simulink model "Snapbot_6leg"  (R2020a)
settings: Solver=FixedStepAuto  StartTime=0.0  StopTime=20  FixedStep=0.001  RelTol=1e-3
PreLoadFcn:
  | startup_Contact_Forces;
InitFcn:
  | SnapbotParameters_6leg;
StopFcn:
  | snapbot_plot;
model workspace (MATLAB code in the model file):
  | % Simscape(TM) Multibody(TM) version: 7.0
  | 
  | % This is a model data file derived from a Simscape Multibody Import XML file using the smimport function.
  | % The data in this file sets the block parameter values in an imported Simscape Multibody model.
  | % For more information on this file, see the smimport function help page in the Simscape Multibody documentation.
  | % You can modify numerical values, but avoid any other changes to this file.
  | % Do not add code to this file. Do not edit the physical units shown in comments.
  | 
  | %%%VariableName:smiData
  | 
  | 
  | %============= RigidTransform =============%
  | 
  | %Initialize the RigidTransform structure array by filling in null values.
  | smiData.RigidTransform(41).translation = [0.0 0.0 0.0];
  | smiData.RigidTransform(41).angle = 0.0;
  | smiData.RigidTransform(41).axis = [0.0 0.0 0.0];
  | smiData.RigidTransform(41).ID = '';
  | 
  | %Translation Method - Cartesian
  | %Rotation Method - Arbitrary Axis
  | smiData.RigidTransform(1).translation = [0 0 3.5000000000000031];  % mm
  | smiData.RigidTransform(1).angle = 0;  % rad
  | smiData.RigidTransform(1).axis = [0 0 0];
  | smiData.RigidTransform(1).ID = 'B[Leg_Assembly_Y-P:Leg_part_01_yaw-1:-:Leg_Assembly_Y-P:v4_Hyb_X-430_IDLE_uncut-1]';
  | 
  | %Translation Method - Cartesian
  | %Rotation Method - Arbitrary Axis
  | smiData.RigidTransform(2).translation = [1.7377765892945298e-13 -35.249999999999865 -4.1211478674085811e-13];  % mm
  | smiData.RigidTransform(2).angle = 3.1415926535897931;  % rad
  | smiData.RigidTransform(2).axis = [3.9252311467098009e-17 -0.70710678118654757 -0.70710678118654746];
  | smiData.RigidTransform(2).ID = 'F[Leg_Assembly_Y-P:Leg_part_01_yaw-1:-:Leg_Assembly_Y-P:v4_Hyb_X-430_IDLE_uncut-1]';
  | 
  | %Translation Method - Cartesian
  | %Rotation Method - Arbitrary Axis
  | smiData.RigidTransform(3).translation = [18.999999999999996 0 -21.500000000000004];  % mm
  | smiData.RigidTransform(3).angle = 2.0943951023931957;  % rad
  | smiData.RigidTransform(3).axis = [0.57735026918962562 0.57735026918962584 0.57735026918962584];
  | smiData.RigidTransform(3).ID = 'B[Leg_Assembly_Y-P:Leg_part_02_Yaw-1:-:Leg_Assembly_Y-P:v4_Hyb_X-430_IDLE_uncut-1]';
  | 
  | %Translation Method - Cartesian
  | %Rotation Method - Arbitrary Axis
  | smiData.RigidTransform(4).translation = [-2.7613467068476893e-12 6.9988459472369868e-13 19];  % mm
  | smiData.RigidTransform(4).angle = 4.7102773760513248e-16;  % rad
  | smiData.RigidTransform(4).axis = [-0.94280904158206347 0.3333333333333332 -7.4014868308343741e-17];
  | smiData.RigidTransform(4).ID = 'F[Leg_Assembly_Y-P:Leg_part_02_Yaw-1:-:Leg_Assembly_Y-P:v4_Hyb_X-430_IDLE_uncut-1]';
  | 
  | %Translation Method - Cartesian
  | %Rotation Method - Arbitrary Axis
  | smiData.RigidTransform(5).translation = [8.3000000000000025 6.0000000000000009 -1.5000000000000013];  % mm
  | smiData.RigidTransform(5).angle = 3.1415926535897931;  % rad
  | smiData.RigidTransform(5).axis = [1 0 0];
  | smiData.RigidTransform(5).ID = 'B[Leg_Assembly_Y-P:Leg_part_02_Yaw-1:-:Leg_Assembly_Y-P:v4_Hyb_X-430_IDLE_uncut-2]';
  | 
  | %Translation Method - Cartesian
  | %Rotation Method - Arbitrary Axis
  | smiData.RigidTransform(6).translation = [-8.0000000000000853 -36.749999999999993 6.0000000000000142];  % mm
  | smiData.RigidTransform(6).angle = 3.1415926535897931;  % rad
  | smiData.RigidTransform(6).axis = [5.5511151231257827e-17 0.70710678118654757 -0.70710678118654746];
  | smiData.RigidTransform(6).ID = 'F[Leg_Assembly_Y-P:Leg_part_02_Yaw-1:-:Leg_Assembly_Y-P:v4_Hyb_X-430_IDLE_uncut-2]';
  | 
  | %Translation Method - Cartesian
  | %Rotation Method - Arbitrary Axis
  | smiData.RigidTransform(7).translation = [-5.7500000000000053 17.749999999999996 20.999999999999993];  % mm
  | smiData.RigidTransform(7).angle = 2.0943951023931953;  % rad
  | smiData.RigidTransform(7).axis = [0.57735026918962584 -0.57735026918962584 0.57735026918962584];
  | smiData.RigidTransform(7).ID = 'B[Leg_Assembly_Y-P:Leg_part_03-1:-:Leg_Assembly_Y-P:v4_Hyb_X-430_IDLE_uncut-2]';
  | 
  | %Translation Method - Cartesian
  | %Rotation Method - Arbitrary Axis
  | smiData.RigidTransform(8).translation = [-17.75000000000005 -4.0000000000015383 6.000000000000135];  % mm
  | smiData.RigidTransform(8).angle = 2.0943951023931953;  % rad
  | smiData.RigidTransform(8).axis = [0.57735026918962562 0.57735026918962584 0.57735026918962595];
  | smiData.RigidTransform(8).ID = 'F[Leg_Assembly_Y-P:Leg_part_03-1:-:Leg_Assembly_Y-P:v4_Hyb_X-430_IDLE_uncut-2]';
  | 
  | %Translation Method - Cartesian
  | %Rotation Method - Arbitrary Axis
  | smiData.RigidTransform(9).translation = [47.999999999999986 0 0];  % mm
  | smiData.RigidTransform(9).angle = 2.0943951023931953;  % rad
  | smiData.RigidTransform(9).axis = [-0.57735026918962584 -0.57735026918962584 0.57735026918962584];
  | smiData.RigidTransform(9).ID = 'B[Leg_Assembly_Y-P:Leg_part_04-1:-:Leg_Assembly_Y-P:v4_Hyb_X-430_IDLE_uncut-2]';
  | 
  | %Translation Method - Cartesian
  | %Rotation Method - Arbitrary Axis
  | smiData.RigidTransform(10).translation = [-1.2789769243681803e-12 1.5383250229206169e-12 24.000000000000025];  % mm
  | smiData.RigidTransform(10).angle = 3.1415926535897931;  % rad
  | smiData.RigidTransform(10).axis = [1 2.1382117680737565e-50 2.7755575615628914e-17];
  | smiData.RigidTransform(10).ID = 'F[Leg_Assembly_Y-P:Leg_part_04-1:-:Leg_Assembly_Y-P:v4_Hyb_X-430_IDLE_uncut-2]';
  | 
  | %Translation Method - Cartesian
  | %Rotation Method - Arbitrary Axis
  | smiData.RigidTransform(11).translation = [21.999999999999993 6.0000000000000053 -15.000000000000004];  % mm
  | smiData.RigidTransform(11).angle = 0;  % rad
  | smiData.RigidTransform(11).axis = [0 0 0];
  | smiData.RigidTransform(11).ID = 'B[Leg_Assembly_Y-P:Leg_part_03-1:-:Leg_Assembly_Y-P:Leg_part_06-1]';
  | 
  | %Translation Method - Cartesian
  | %Rotation Method - Arbitrary Axis
  | smiData.RigidTransform(12).translation = [-25.499999999999993 -6.4730443227745127e-12 -47.429999999998479];  % mm
  | smiData.RigidTransform(12).angle = 2.0943951023931953;  % rad
  | smiData.RigidTransform(12).axis = [0.57735026918962584 0.57735026918962584 0.57735026918962584];
  | smiData.RigidTransform(12).ID = 'F[Leg_Assembly_Y-P:Leg_part_03-1:-:Leg_Assembly_Y-P:Leg_part_06-1]';
  | 
  | %Translation Method - Cartesian
  | %Rotation Method - Arbitrary Axis
  | smiData.RigidTransform(13).translation = [18.500000000000004 0 0];  % mm
  | smiData.RigidTransform(13).angle = 2.0943951023931957;  % rad
  | smiData.RigidTransform(13).axis = [-0.57735026918962584 -0.57735026918962573 0.57735026918962573];
  | smiData.RigidTransform(13).ID = 'B[Leg_Assembly_Y-P:Leg_part_05-1:-:Leg_Assembly_Y-P:Leg_part_04-1]';
  | 
  | %Translation Method - Cartesian
  | %Rotation Method - Arbitrary Axis
  | smiData.RigidTransform(14).translation = [5.4999999999999645 -6.1227943166086393e-12 -59.999999999989711];  % mm
  | smiData.RigidTransform(14).angle = 2.0943951023931953;  % rad
  | smiData.RigidTransform(14).axis = [0.57735026918962584 0.57735026918962584 0.57735026918962584];
  | smiData.RigidTransform(14).ID = 'F[Leg_Assembly_Y-P:Leg_part_05-1:-:Leg_Assembly_Y-P:Leg_part_04-1]';
  | 
  | %Translation Method - Cartesian
  | %Rotation Method - Arbitrary Axis
  | smiData.RigidTransform(15).translation = [-4.5000000000000009 25 0];  % mm
  | smiData.RigidTransform(15).angle = 2.0943951023931953;  % rad
  | smiData.RigidTransform(15).axis = [-0.57735026918962584 -0.57735026918962584 0.57735026918962584];
  | smiData.RigidTransform(15).ID = 'B[Leg_Assembly_Y-P:Leg_part_05-1:-:Leg_Assembly_Y-P:Leg_part_06-1]';
  | 
  | %Translation Method - Cartesian
  | %Rotation Method - Arbitrary Axis
  | smiData.RigidTransform(16).translation = [8.9999999999998792 1.925328508647566e-12 -7.783518711315191e-13];  % mm
  | smiData.RigidTransform(16).angle = 2.0943951023931957;  % rad
  | smiData.RigidTransform(16).axis = [0.57735026918962584 0.57735026918962584 0.57735026918962562];
  | smiData.RigidTransform(16).ID = 'F[Leg_Assembly_Y-P:Leg_part_05-1:-:Leg_Assembly_Y-P:Leg_part_06-1]';
  | 
  | %Translation Method - Cartesian
  | %Rotation Method - Arbitrary Axis
  | smiData.RigidTransform(17).translation = [-29.14813879243771 31.324765133364547 -50.486057334570816];  % mm
  | smiData.RigidTransform(17).angle = 0.85969556486762932;  % rad
  | smiData.RigidTransform(17).axis = [-0.88342402684813537 0.43430848851138709 -0.17589236934665334];
  | smiData.RigidTransform(17).ID = 'B[Body_Frame-2:-:cover_IMU-1]';
  | 
  | %Translation Method - Cartesian
  | %Rotation Method - Arbitrary Axis
  | smiData.RigidTransform(18).translation = [-29.148138792437663 -3.675234866635499 -50.486057334570852];  % mm
  | smiData.RigidTransform(18).angle = 0.85969556486762932;  % rad
  | smiData.RigidTransform(18).axis = [-0.88342402684813526 0.43430848851138698 -0.17589236934665331];
  | smiData.RigidTransform(18).ID = 'F[Body_Frame-2:-:cover_IMU-1]';
  | 
  | %Translation Method - Cartesian
  | %Rotation Method - Arbitrary Axis
  | smiData.RigidTransform(19).translation = [-60.000000000000043 24.02083948120934 0];  % mm
  | smiData.RigidTransform(19).angle = 2.5346467848844187;  % rad
  | smiData.RigidTransform(19).axis = [-0.31314561301497384 -0.67154293423781708 0.67154293423781863];
  | smiData.RigidTransform(19).ID = 'B[Body_Frame-2:-:Leg_Assembly_Y-P-5:Leg_part_01_yaw-1]';
  | 
  | %Translation Method - Cartesian
  | %Rotation Method - Arbitrary Axis
  | smiData.RigidTransform(20).translation = [3.7154631030277672e-13 16.020839481209393 -21.000000000000213];  % mm
  | smiData.RigidTransform(20).angle = 1.6880425449503949;  % rad
  | smiData.RigidTransform(20).axis = [0.32361557711818967 -0.32361557711818179 0.88912649071598759];
  | smiData.RigidTransform(20).ID = 'F[Body_Frame-2:-:Leg_Assembly_Y-P-5:Leg_part_01_yaw-1]';
  | 
  | %Translation Method - Cartesian
  | %Rotation Method - Arbitrary Axis
  | smiData.RigidTransform(21).translation = [-17.984370389093243 16.010419740604632 -58.898751217406307];  % mm
  | smiData.RigidTransform(21).angle = 2.5668813081404753;  % rad
  | smiData.RigidTransform(21).axis = [-0.54469904781872214 -0.67552162020226258 0.49696427230203144];
  | smiData.RigidTransform(21).ID = 'B[Body_Frame-2:-:Leg_Assembly_Y-P-4:Leg_part_01_yaw-1]';
  | 
  | %Translation Method - Cartesian
  | %Rotation Method - Arbitrary Axis
  | smiData.RigidTransform(22).translation = [-13.874453980679904 8.0104197406047888 -21.000000000000171];  % mm
  | smiData.RigidTransform(22).angle = 1.5933089052267559;  % rad
  | smiData.RigidTransform(22).axis = [0.45474157432660411 0.14837486987203785 0.87817708838788178];
  | smiData.RigidTransform(22).ID = 'F[Body_Frame-2:-:Leg_Assembly_Y-P-4:Leg_part_01_yaw-1]';
  | 
  | %Translation Method - Cartesian
  | %Rotation Method - Arbitrary Axis
  | smiData.RigidTransform(23).translation = [0 50 0];  % mm
  | smiData.RigidTransform(23).angle = 2.0943951023931953;  % rad
  | smiData.RigidTransform(23).axis = [-0.57735026918962584 -0.57735026918962584 -0.57735026918962584];
  | smiData.RigidTransform(23).ID = 'B[floor-1:-:]';
  | 
  | %Translation Method - Cartesian
  | %Rotation Method - Arbitrary Axis
  | smiData.RigidTransform(24).translation = [0 -7.1054273576010019e-15 0];  % mm
  | smiData.RigidTransform(24).angle = 3.1415926535897931;  % rad
  | smiData.RigidTransform(24).axis = [0.70710678118654757 0.70710678118654757 -5.5511151231257839e-17];
  | smiData.RigidTransform(24).ID = 'F[floor-1:-:]';
  | 
  | %Translation Method - Cartesian
  | %Rotation Method - Arbitrary Axis
  | smiData.RigidTransform(25).translation = [29.999999999999982 24.02083948120934 -51.961524227066384];  % mm
  | smiData.RigidTransform(25).angle = 2.3875525638501713;  % rad
  | smiData.RigidTransform(25).axis = [0.97769691900991618 0.078837114487629617 0.19466238449629064];
  | smiData.RigidTransform(25).ID = 'B[Body_Frame-2:-:Leg_Assembly_Y-P-3:Leg_part_01_yaw-1]';
  | 
  | %Translation Method - Cartesian
  | %Rotation Method - Arbitrary Axis
  | smiData.RigidTransform(26).translation = [-4.3698378249246161e-13 16.020839481209286 -20.999999999999972];  % mm
  | smiData.RigidTransform(26).angle = 2.8078721686781996;  % rad
  | smiData.RigidTransform(26).axis = [0.061302152168850967 -0.34137689046920633 0.93792529808777547];
  | smiData.RigidTransform(26).ID = 'F[Body_Frame-2:-:Leg_Assembly_Y-P-3:Leg_part_01_yaw-1]';
  | 
  | %Translation Method - Cartesian
  | %Rotation Method - Arbitrary Axis
  | smiData.RigidTransform(27).translation = [30.000000000000536 24.02083948120934 51.961524227066057];  % mm
  | smiData.RigidTransform(27).angle = 0.85969556486763532;  % rad
  | smiData.RigidTransform(27).axis = [0.88342402684813182 0.43430848851139292 0.17589236934665639];
  | smiData.RigidTransform(27).ID = 'B[Body_Frame-2:-:Leg_Assembly_Y-P-2:Leg_part_01_yaw-1]';
  | 
  | %Translation Method - Cartesian
  | %Rotation Method - Arbitrary Axis
  | smiData.RigidTransform(28).translation = [5.6843418860808015e-14 16.020839481209322 -21.000000000000114];  % mm
  | smiData.RigidTransform(28).angle = 0.7800553012765955;  % rad
  | smiData.RigidTransform(28).axis = [0.88538441591605921 -0.15899134272919926 0.43682512403723389];
  | smiData.RigidTransform(28).ID = 'F[Body_Frame-2:-:Leg_Assembly_Y-P-2:Leg_part_01_yaw-1]';
  | 
  | %Translation Method - Cartesian
  | %Rotation Method - Arbitrary Axis
  | smiData.RigidTransform(29).translation = [0 16.020839481209414 -20.999999999999996];  % mm
  | smiData.RigidTransform(29).angle = 2.4434609527920594;  % rad
  | smiData.RigidTransform(29).axis = [-1 -2.3686015843339707e-16 6.5076793686420059e-16];
  | smiData.RigidTransform(29).ID = 'B[Leg_Assembly_Y-P-1:Leg_part_01_yaw-1:-:Body_Frame-2]';
  | 
  | %Translation Method - Cartesian
  | %Rotation Method - Arbitrary Axis
  | smiData.RigidTransform(30).translation = [-29.999999999999154 24.020839481209457 51.961524227066796];  % mm
  | smiData.RigidTransform(30).angle = 2.4682098215588208;  % rad
  | smiData.RigidTransform(30).axis = [-0.96166828182989805 -0.093787209197188054 -0.25767823950294];
  | smiData.RigidTransform(30).ID = 'F[Leg_Assembly_Y-P-1:Leg_part_01_yaw-1:-:Body_Frame-2]';
  | 
  | %Translation Method - Cartesian
  | %Rotation Method - Arbitrary Axis
  | smiData.RigidTransform(31).translation = [58.296277584874844 -3.6752348666354435 0];  % mm
  | smiData.RigidTransform(31).angle = 1.750366012803156;  % rad
  | smiData.RigidTransform(31).axis = [0.83481712947898612 0.38928162063502714 0.38928162063502642];
  | smiData.RigidTransform(31).ID = 'B[cover-2:-:Body_Frame-2]';
  | 
  | %Translation Method - Cartesian
  | %Rotation Method - Arbitrary Axis
  | smiData.RigidTransform(32).translation = [-58.296277584874161 -15.324765133364131 2.3909763058327371e-12];  % mm
  | smiData.RigidTransform(32).angle = 2.534646784884413;  % rad
  | smiData.RigidTransform(32).axis = [0.31314561301496746 -0.67154293423781519 -0.67154293423782341];
  | smiData.RigidTransform(32).ID = 'F[cover-2:-:Body_Frame-2]';
  | 
  | %Translation Method - Cartesian
  | %Rotation Method - Arbitrary Axis
  | smiData.RigidTransform(33).translation = [60.000000000000043 24.02083948120934 0];  % mm
  | smiData.RigidTransform(33).angle = 1.7503660128031577;  % rad
  | smiData.RigidTransform(33).axis = [0.83481712947898612 0.38928162063502897 0.38928162063502469];
  | smiData.RigidTransform(33).ID = 'B[Body_Frame-2:-:Leg_Assembly_Y-P-6:Leg_part_01_yaw-1]';
  | 
  | %Translation Method - Cartesian
  | %Rotation Method - Arbitrary Axis
  | smiData.RigidTransform(34).translation = [5.3069536461860958e-13 16.020839481209272 -21.000000000000171];  % mm
  | smiData.RigidTransform(34).angle = 1.6880425449503949;  % rad
  | smiData.RigidTransform(34).axis = [0.32361557711818967 -0.32361557711818206 0.88912649071598748];
  | smiData.RigidTransform(34).ID = 'F[Body_Frame-2:-:Leg_Assembly_Y-P-6:Leg_part_01_yaw-1]';
  | 
  | %Translation Method - Cartesian
  | %Rotation Method - Arbitrary Axis
  | smiData.RigidTransform(35).translation = [-0.53570167355018905 37.318511693782639 54.569829435763872];  % mm
  | smiData.RigidTransform(35).angle = 0;  % rad
  | smiData.RigidTransform(35).axis = [0 0 0];
  | smiData.RigidTransform(35).ID = 'AssemblyGround[Leg_Assembly_Y-P-1:Leg_part_01_yaw-1]';
  | 
  | %Translation Method - Cartesian
  | %Rotation Method - Arbitrary Axis
  | smiData.RigidTransform(36).translation = [-0.53570167355018106 37.318511693782625 54.569829435763914];  % mm
  | smiData.RigidTransform(36).angle = 0;  % rad
  | smiData.RigidTransform(36).axis = [0 0 0];
  | smiData.RigidTransform(36).ID = 'AssemblyGround[Leg_Assembly_Y-P-2:Leg_part_01_yaw-1]';
  | 
  | %Translation Method - Cartesian
  | %Rotation Method - Arbitrary Axis
  | smiData.RigidTransform(37).translation = [-0.53570167355018228 37.318511693782625 54.569829435763921];  % mm
  | smiData.RigidTransform(37).angle = 0;  % rad
  | smiData.RigidTransform(37).axis = [0 0 0];
  | smiData.RigidTransform(37).ID = 'AssemblyGround[Leg_Assembly_Y-P-3:Leg_part_01_yaw-1]';
  | 
  | %Translation Method - Cartesian
  | %Rotation Method - Arbitrary Axis
  | smiData.RigidTransform(38).translation = [-0.53570167355018561 37.318511693782625 54.569829435763857];  % mm
  | smiData.RigidTransform(38).angle = 0;  % rad
  | smiData.RigidTransform(38).axis = [0 0 0];
  | smiData.RigidTransform(38).ID = 'AssemblyGround[Leg_Assembly_Y-P-5:Leg_part_01_yaw-1]';
  | 
  | %Translation Method - Cartesian
  | %Rotation Method - Arbitrary Axis
  | smiData.RigidTransform(39).translation = [-0.53570167355018039 37.318511693782639 54.569829435763864];  % mm
  | smiData.RigidTransform(39).angle = 0;  % rad
  | smiData.RigidTransform(39).axis = [0 0 0];
  | smiData.RigidTransform(39).ID = 'AssemblyGround[Leg_Assembly_Y-P-4:Leg_part_01_yaw-1]';
  | 
  | %Translation Method - Cartesian
  | %Rotation Method - Arbitrary Axis
  | smiData.RigidTransform(40).translation = [-0.53570167355017972 37.318511693782597 54.569829435763886];  % mm
  | smiData.RigidTransform(40).angle = 0;  % rad
  | smiData.RigidTransform(40).axis = [0 0 0];
  | smiData.RigidTransform(40).ID = 'AssemblyGround[Leg_Assembly_Y-P-6:Leg_part_01_yaw-1]';
  | 
  | %Translation Method - Cartesian
  | %Rotation Method - Arbitrary Axis
  | smiData.RigidTransform(41).translation = [1.1102230246251479e-12 3.2151978216727191e-12 132.50000000000026];  % mm
  | smiData.RigidTransform(41).angle = 2.0943951023931957;  % rad
  | smiData.RigidTransform(41).axis = [0.57735026918962573 -0.57735026918962562 -0.57735026918962573];
  | smiData.RigidTransform(41).ID = 'SixDofRigidTransform[Body_Frame-2]';
  | 
  | 
  | %============= Solid =============%
  | %Center of Mass (CoM) %Moments of Inertia (MoI) %Product of Inertia (PoI)
  | 
  | %Initialize the Solid structure array by filling in null values.
  | smiData.Solid(11).mass = 0.0;
  | smiData.Solid(11).CoM = [0.0 0.0 0.0];
  | smiData.Solid(11).MoI = [0.0 0.0 0.0];
  | smiData.Solid(11).PoI = [0.0 0.0 0.0];
  | smiData.Solid(11).color = [0.0 0.0 0.0];
  | smiData.Solid(11).opacity = 0.0;
  | smiData.Solid(11).ID = '';
  | 
  | %Inertia Type - Custom
  | %Visual Properties - Simple
  | smiData.Solid(1).mass = 49.999999999999993;  % kg
  | smiData.Solid(1).CoM = [0 25.000000000000004 0];  % mm
  | smiData.Solid(1).MoI = [4177083.333333333 8333333.333333334 4177083.333333333];  % kg*mm^2
  | smiData.Solid(1).PoI = [0 -7.6327832942979522e-10 0];  % kg*mm^2
  | smiData.Solid(1).color = [0.792156862745098 0.81960784313725488 0.93333333333333335];
  | smiData.Solid(1).opacity = 1;
  | smiData.Solid(1).ID = 'floor*:*Default';
  | 
  | %Inertia Type - Custom
  | %Visual Properties - Simple
  | smiData.Solid(2).mass = 0.069142856834278052;  % kg
  | smiData.Solid(2).CoM = [-6.5363888180793326e-08 8.0286872966298493 -0.84505300940729178];  % mm
  | smiData.Solid(2).MoI = [133.83817269769426 248.31514966138255 134.30804068565405];  % kg*mm^2
  | smiData.Solid(2).PoI = [0.10611953301327832 3.6362614035336834e-07 -3.5551676350249992e-07];  % kg*mm^2
  | smiData.Solid(2).color = [0.75294117647058822 0.75294117647058822 0.75294117647058822];
  | smiData.Solid(2).opacity = 1;
  | smiData.Solid(2).ID = 'Body_Frame*:*Default';
  | 
  | %Inertia Type - Custom
  | %Visual Properties - Simple
  | smiData.Solid(3).mass = 0.011990679618999286;  % kg
  | smiData.Solid(3).CoM = [0.00075299564053924969 1.2041866129100636 0.00017910245223251136];  % mm
  | smiData.Solid(3).MoI = [12.311205329208734 24.493353479322121 12.311271128519959];  % kg*mm^2
  | smiData.Solid(3).PoI = [1.0644747991253964e-05 -8.6961826208665648e-05 1.824565847520757e-05];  % kg*mm^2
  | smiData.Solid(3).color = [0.792156862745098 0.81960784313725488 0.93333333333333335];
  | smiData.Solid(3).opacity = 1;
  | smiData.Solid(3).ID = 'cover_IMU*:*Default';
  | 
  | %Inertia Type - Custom
  | %Visual Properties - Simple
  | smiData.Solid(4).mass = 0.043283962506312126;  % kg
  | smiData.Solid(4).CoM = [0 -11.629154441205349 0.58622657822569368];  % mm
  | smiData.Solid(4).MoI = [11.945660403890635 6.9373449472329325 10.473897647404552];  % kg*mm^2
  | smiData.Solid(4).PoI = [-0.010479195470367065 0 0];  % kg*mm^2
  | smiData.Solid(4).color = [0.50196078431372548 0.50196078431372548 0.50196078431372548];
  | smiData.Solid(4).opacity = 1;
  | smiData.Solid(4).ID = 'v4_Hyb_X-430_IDLE_uncut*:*Default';
  | 
  | %Inertia Type - Custom
  | %Visual Properties - Simple
  | smiData.Solid(5).mass = 0.015928924279537779;  % kg
  | smiData.Solid(5).CoM = [5.5724533955433566 0.60923661115773331 14.965495324586268];  % mm
  | smiData.Solid(5).MoI = [6.7178267454302487 3.3961346093070595 5.3516535264104634];  % kg*mm^2
  | smiData.Solid(5).PoI = [0.0029589860947701013 0.0090414356066351453 -0.14024072638650098];  % kg*mm^2
  | smiData.Solid(5).color = [0.50196078431372548 1 1];
  | smiData.Solid(5).opacity = 1;
  | smiData.Solid(5).ID = 'Leg_part_03*:*Default';
  | 
  | %Inertia Type - Custom
  | %Visual Properties - Simple
  | smiData.Solid(6).mass = 0.01532092516699415;  % kg
  | smiData.Solid(6).CoM = [23.99999768920209 1.2961678062824165 -35.100094443023529];  % mm
  | smiData.Solid(6).MoI = [10.22123294031608 14.203511884952173 5.0157635391797415];  % kg*mm^2
  | smiData.Solid(6).PoI = [0.58071119483444811 9.2473756048793079e-07 -5.4914041407587592e-06];  % kg*mm^2
  | smiData.Solid(6).color = [1 0.38823529411764707 0.41960784313725491];
  | smiData.Solid(6).opacity = 1;
  | smiData.Solid(6).ID = 'Leg_part_04*:*Default';
  | 
  | %Inertia Type - Custom
  | %Visual Properties - Simple
  | smiData.Solid(7).mass = 0.022715083434313933;  % kg
  | smiData.Solid(7).CoM = [4.7495790018670679e-05 -5.2914882898767052e-07 0.5165057921701256];  % mm
  | smiData.Solid(7).MoI = [6.0201227624572091 7.3567997591054697 10.813457729002581];  % kg*mm^2
  | smiData.Solid(7).PoI = [5.9445977509619064e-08 -2.8721317734098932e-06 -2.6844578174760262e-06];  % kg*mm^2
  | smiData.Solid(7).color = [0.027450980392156862 1 0.027450980392156862];
  | smiData.Solid(7).opacity = 1;
  | smiData.Solid(7).ID = 'Leg_part_02_Yaw*:*Default';
  | 
  | %Inertia Type - Custom
  | %Visual Properties - Simple
  | smiData.Solid(8).mass = 0.022008322051922449;  % kg
  | smiData.Solid(8).CoM = [-0.00020078562165670621 -0.086645709821861094 -7.0226871847428578];  % mm
  | smiData.Solid(8).MoI = [6.5441760223709542 5.8120654403371752 5.5882327823375002];  % kg*mm^2
  | smiData.Solid(8).PoI = [-0.022603449848346446 -3.352686832653925e-05 -5.8881839756598183e-05];  % kg*mm^2
  | smiData.Solid(8).color = [0.9882352941176471 0.73725490196078436 0.51764705882352935];
  | smiData.Solid(8).opacity = 1;
  | smiData.Solid(8).ID = 'Leg_part_01_yaw*:*Default';
  | 
  | %Inertia Type - Custom
  | %Visual Properties - Simple
  | smiData.Solid(9).mass = 0.014765646142892632;  % kg
  | smiData.Solid(9).CoM = [1.2086758172751703e-05 38.516029865216908 1.6102137958750217e-05];  % mm
  | smiData.Solid(9).MoI = [11.438112427079185 0.88080259805912509 11.92628093115035];  % kg*mm^2
  | smiData.Solid(9).PoI = [1.3310978313730002e-06 5.7966270342722696e-06 1.0118234103070852e-06];  % kg*mm^2
  | smiData.Solid(9).color = [0.039215686274509803 0.63137254901960782 0.90588235294117647];
  | smiData.Solid(9).opacity = 1;
  | smiData.Solid(9).ID = 'Leg_part_05*:*Default';
  | 
  | %Inertia Type - Custom
  | %Visual Properties - Simple
  | smiData.Solid(10).mass = 0.0061788723822202929;  % kg
  | smiData.Solid(10).CoM = [4.2543802409912495 -4.630092097224253 -20.149819352752836];  % mm
  | smiData.Solid(10).MoI = [2.2893274182864181 2.0053458866812131 0.35993641872183119];  % kg*mm^2
  | smiData.Solid(10).PoI = [0.20173149787382888 -0.0054107076234519427 0.0070268738351532299];  % kg*mm^2
  | smiData.Solid(10).color = [0.8666666666666667 0.46666666666666667 0.094117647058823528];
  | smiData.Solid(10).opacity = 1;
  | smiData.Solid(10).ID = 'Leg_part_06*:*Default';
  | 
  | %Inertia Type - Custom
  | %Visual Properties - Simple
  | smiData.Solid(11).mass = 0.011859040673008395;  % kg
  | smiData.Solid(11).CoM = [9.2568952008978674e-05 1.1917658906433921 -6.4265217793451617e-05];  % mm
  | smiData.Solid(11).MoI = [12.336903139260397 24.543407766477518 12.33692406602713];  % kg*mm^2
  | smiData.Solid(11).PoI = [1.0093449366405608e-06 3.0788090303879734e-05 -1.064469578393175e-06];  % kg*mm^2
  | smiData.Solid(11).color = [0.792156862745098 0.81960784313725488 0.93333333333333335];
  | smiData.Solid(11).opacity = 1;
  | smiData.Solid(11).ID = 'cover*:*Default';
  | 
  | 
  | %============= Joint =============%
  | %X Revolute Primitive (Rx) %Y Revolute Primitive (Ry) %Z Revolute Primitive (Rz)
  | %X Prismatic Primitive (Px) %Y Prismatic Primitive (Py) %Z Prismatic Primitive (Pz) %Spherical Primitive (S)
  | %Constant Velocity Primitive (CV) %Lead Screw Primitive (LS)
  | %Position Target (Pos)
  | 
  | %Initialize the CylindricalJoint structure array by filling in null values.
  | smiData.CylindricalJoint(6).Rz.Pos = 0.0;
  | smiData.CylindricalJoint(6).Pz.Pos = 0.0;
  | smiData.CylindricalJoint(6).ID = '';
  | 
  | %This joint has been chosen as a cut joint. Simscape Multibody treats cut joints as algebraic constraints to solve closed kinematic loops. The imported model does not use the state target data for this joint.
  | smiData.CylindricalJoint(1).Rz.Pos = -40.005411760834768;  % deg
  | smiData.CylindricalJoint(1).Pz.Pos = 0;  % mm
  | smiData.CylindricalJoint(1).ID = '[Leg_Assembly_Y-P-1:Leg_part_05-1:-:Leg_Assembly_Y-P-1:Leg_part_06-1]';
  | 
  | %This joint has been chosen as a cut joint. Simscape Multibody treats cut joints as algebraic constraints to solve closed kinematic loops. The imported model does not use the state target data for this joint.
  | smiData.CylindricalJoint(2).Rz.Pos = -40.005411760834768;  % deg
  | smiData.CylindricalJoint(2).Pz.Pos = 0;  % mm
  | smiData.CylindricalJoint(2).ID = '[Leg_Assembly_Y-P-2:Leg_part_05-1:-:Leg_Assembly_Y-P-2:Leg_part_06-1]';
  | 
  | %This joint has been chosen as a cut joint. Simscape Multibody treats cut joints as algebraic constraints to solve closed kinematic loops. The imported model does not use the state target data for this joint.
  | smiData.CylindricalJoint(3).Rz.Pos = -40.005411760834768;  % deg
  | smiData.CylindricalJoint(3).Pz.Pos = 0;  % mm
  | smiData.CylindricalJoint(3).ID = '[Leg_Assembly_Y-P-3:Leg_part_05-1:-:Leg_Assembly_Y-P-3:Leg_part_06-1]';
  | 
  | %This joint has been chosen as a cut joint. Simscape Multibody treats cut joints as algebraic constraints to solve closed kinematic loops. The imported model does not use the state target data for this joint.
  | smiData.CylindricalJoint(4).Rz.Pos = -40.005411760834768;  % deg
  | smiData.CylindricalJoint(4).Pz.Pos = 0;  % mm
  | smiData.CylindricalJoint(4).ID = '[Leg_Assembly_Y-P-5:Leg_part_05-1:-:Leg_Assembly_Y-P-5:Leg_part_06-1]';
  | 
  | %This joint has been chosen as a cut joint. Simscape Multibody treats cut joints as algebraic constraints to solve closed kinematic loops. The imported model does not use the state target data for this joint.
  | smiData.CylindricalJoint(5).Rz.Pos = -40.005411760834761;  % deg
  | smiData.CylindricalJoint(5).Pz.Pos = 0;  % mm
  | smiData.CylindricalJoint(5).ID = '[Leg_Assembly_Y-P-4:Leg_part_05-1:-:Leg_Assembly_Y-P-4:Leg_part_06-1]';
  | 
  | %This joint has been chosen as a cut joint. Simscape Multibody treats cut joints as algebraic constraints to solve closed kinematic loops. The imported model does not use the state target data for this joint.
  | smiData.CylindricalJoint(6).Rz.Pos = -40.005411760834754;  % deg
  | smiData.CylindricalJoint(6).Pz.Pos = 0;  % mm
  | smiData.CylindricalJoint(6).ID = '[Leg_Assembly_Y-P-6:Leg_part_05-1:-:Leg_Assembly_Y-P-6:Leg_part_06-1]';
  | 
  | 
  | %Initialize the RevoluteJoint structure array by filling in null values.
  | smiData.RevoluteJoint(30).Rz.Pos = 0.0;
  | smiData.RevoluteJoint(30).ID = '';
  | 
  | smiData.RevoluteJoint(1).Rz.Pos = -4.0057075510311417e-30;  % deg
  | smiData.RevoluteJoint(1).ID = '[Leg_Assembly_Y-P-1:Leg_part_02_Yaw-1:-:Leg_Assembly_Y-P-1:v4_Hyb_X-430_IDLE_uncut-1]';
  | 
  | smiData.RevoluteJoint(2).Rz.Pos = -89.999999999999972;  % deg
  | smiData.RevoluteJoint(2).ID = '[Leg_Assembly_Y-P-1:Leg_part_03-1:-:Leg_Assembly_Y-P-1:v4_Hyb_X-430_IDLE_uncut-2]';
  | 
  | smiData.RevoluteJoint(3).Rz.Pos = 180;  % deg
  | smiData.RevoluteJoint(3).ID = '[Leg_Assembly_Y-P-1:Leg_part_04-1:-:Leg_Assembly_Y-P-1:v4_Hyb_X-430_IDLE_uncut-2]';
  | 
  | smiData.RevoluteJoint(4).Rz.Pos = -130.80925683646447;  % deg
  | smiData.RevoluteJoint(4).ID = '[Leg_Assembly_Y-P-1:Leg_part_03-1:-:Leg_Assembly_Y-P-1:Leg_part_06-1]';
  | 
  | smiData.RevoluteJoint(5).Rz.Pos = -179.19615492437035;  % deg
  | smiData.RevoluteJoint(5).ID = '[Leg_Assembly_Y-P-1:Leg_part_05-1:-:Leg_Assembly_Y-P-1:Leg_part_04-1]';
  | 
  | smiData.RevoluteJoint(6).Rz.Pos = 8.9959671327898901e-15;  % deg
  | smiData.RevoluteJoint(6).ID = '[Leg_Assembly_Y-P-2:Leg_part_02_Yaw-1:-:Leg_Assembly_Y-P-2:v4_Hyb_X-430_IDLE_uncut-1]';
  | 
  | smiData.RevoluteJoint(7).Rz.Pos = -90;  % deg
  | smiData.RevoluteJoint(7).ID = '[Leg_Assembly_Y-P-2:Leg_part_03-1:-:Leg_Assembly_Y-P-2:v4_Hyb_X-430_IDLE_uncut-2]';
  | 
  | smiData.RevoluteJoint(8).Rz.Pos = 180;  % deg
  | smiData.RevoluteJoint(8).ID = '[Leg_Assembly_Y-P-2:Leg_part_04-1:-:Leg_Assembly_Y-P-2:v4_Hyb_X-430_IDLE_uncut-2]';
  | 
  | smiData.RevoluteJoint(9).Rz.Pos = -130.80925683646447;  % deg
  | smiData.RevoluteJoint(9).ID = '[Leg_Assembly_Y-P-2:Leg_part_03-1:-:Leg_Assembly_Y-P-2:Leg_part_06-1]';
  | 
  | smiData.RevoluteJoint(10).Rz.Pos = -179.19615492437032;  % deg
  | smiData.RevoluteJoint(10).ID = '[Leg_Assembly_Y-P-2:Leg_part_05-1:-:Leg_Assembly_Y-P-2:Leg_part_04-1]';
  | 
  | smiData.RevoluteJoint(11).Rz.Pos = 8.9959671327898901e-15;  % deg
  | smiData.RevoluteJoint(11).ID = '[Leg_Assembly_Y-P-3:Leg_part_02_Yaw-1:-:Leg_Assembly_Y-P-3:v4_Hyb_X-430_IDLE_uncut-1]';
  | 
  | smiData.RevoluteJoint(12).Rz.Pos = -90;  % deg
  | smiData.RevoluteJoint(12).ID = '[Leg_Assembly_Y-P-3:Leg_part_03-1:-:Leg_Assembly_Y-P-3:v4_Hyb_X-430_IDLE_uncut-2]';
  | 
  | smiData.RevoluteJoint(13).Rz.Pos = 180;  % deg
  | smiData.RevoluteJoint(13).ID = '[Leg_Assembly_Y-P-3:Leg_part_04-1:-:Leg_Assembly_Y-P-3:v4_Hyb_X-430_IDLE_uncut-2]';
  | 
  | smiData.RevoluteJoint(14).Rz.Pos = -130.80925683646447;  % deg
  | smiData.RevoluteJoint(14).ID = '[Leg_Assembly_Y-P-3:Leg_part_03-1:-:Leg_Assembly_Y-P-3:Leg_part_06-1]';
  | 
  | smiData.RevoluteJoint(15).Rz.Pos = -179.19615492437032;  % deg
  | smiData.RevoluteJoint(15).ID = '[Leg_Assembly_Y-P-3:Leg_part_05-1:-:Leg_Assembly_Y-P-3:Leg_part_04-1]';
  | 
  | smiData.RevoluteJoint(16).Rz.Pos = 2.6662089633133513e-13;  % deg
  | smiData.RevoluteJoint(16).ID = '[Leg_Assembly_Y-P-5:Leg_part_02_Yaw-1:-:Leg_Assembly_Y-P-5:v4_Hyb_X-430_IDLE_uncut-1]';
  | 
  | smiData.RevoluteJoint(17).Rz.Pos = -90;  % deg
  | smiData.RevoluteJoint(17).ID = '[Leg_Assembly_Y-P-5:Leg_part_03-1:-:Leg_Assembly_Y-P-5:v4_Hyb_X-430_IDLE_uncut-2]';
  | 
  | smiData.RevoluteJoint(18).Rz.Pos = 180;  % deg
  | smiData.RevoluteJoint(18).ID = '[Leg_Assembly_Y-P-5:Leg_part_04-1:-:Leg_Assembly_Y-P-5:v4_Hyb_X-430_IDLE_uncut-2]';
  | 
  | smiData.RevoluteJoint(19).Rz.Pos = -130.80925683646447;  % deg
  | smiData.RevoluteJoint(19).ID = '[Leg_Assembly_Y-P-5:Leg_part_03-1:-:Leg_Assembly_Y-P-5:Leg_part_06-1]';
  | 
  | smiData.RevoluteJoint(20).Rz.Pos = -179.19615492437032;  % deg
  | smiData.RevoluteJoint(20).ID = '[Leg_Assembly_Y-P-5:Leg_part_05-1:-:Leg_Assembly_Y-P-5:Leg_part_04-1]';
  | 
  | smiData.RevoluteJoint(21).Rz.Pos = 8.9959671327898885e-15;  % deg
  | smiData.RevoluteJoint(21).ID = '[Leg_Assembly_Y-P-4:Leg_part_02_Yaw-1:-:Leg_Assembly_Y-P-4:v4_Hyb_X-430_IDLE_uncut-1]';
  | 
  | smiData.RevoluteJoint(22).Rz.Pos = -89.999999999999972;  % deg
  | smiData.RevoluteJoint(22).ID = '[Leg_Assembly_Y-P-4:Leg_part_03-1:-:Leg_Assembly_Y-P-4:v4_Hyb_X-430_IDLE_uncut-2]';
  | 
  | smiData.RevoluteJoint(23).Rz.Pos = 180;  % deg
  | smiData.RevoluteJoint(23).ID = '[Leg_Assembly_Y-P-4:Leg_part_04-1:-:Leg_Assembly_Y-P-4:v4_Hyb_X-430_IDLE_uncut-2]';
  | 
  | smiData.RevoluteJoint(24).Rz.Pos = -130.80925683646447;  % deg
  | smiData.RevoluteJoint(24).ID = '[Leg_Assembly_Y-P-4:Leg_part_03-1:-:Leg_Assembly_Y-P-4:Leg_part_06-1]';
  | 
  | smiData.RevoluteJoint(25).Rz.Pos = -179.19615492437032;  % deg
  | smiData.RevoluteJoint(25).ID = '[Leg_Assembly_Y-P-4:Leg_part_05-1:-:Leg_Assembly_Y-P-4:Leg_part_04-1]';
  | 
  | smiData.RevoluteJoint(26).Rz.Pos = 2.6348577698622696e-15;  % deg
  | smiData.RevoluteJoint(26).ID = '[Leg_Assembly_Y-P-6:Leg_part_02_Yaw-1:-:Leg_Assembly_Y-P-6:v4_Hyb_X-430_IDLE_uncut-1]';
  | 
  | smiData.RevoluteJoint(27).Rz.Pos = -89.999999999999986;  % deg
  | smiData.RevoluteJoint(27).ID = '[Leg_Assembly_Y-P-6:Leg_part_03-1:-:Leg_Assembly_Y-P-6:v4_Hyb_X-430_IDLE_uncut-2]';
  | 
  | smiData.RevoluteJoint(28).Rz.Pos = 180;  % deg
  | smiData.RevoluteJoint(28).ID = '[Leg_Assembly_Y-P-6:Leg_part_04-1:-:Leg_Assembly_Y-P-6:v4_Hyb_X-430_IDLE_uncut-2]';
  | 
  | smiData.RevoluteJoint(29).Rz.Pos = -130.80925683646447;  % deg
  | smiData.RevoluteJoint(29).ID = '[Leg_Assembly_Y-P-6:Leg_part_03-1:-:Leg_Assembly_Y-P-6:Leg_part_06-1]';
  | 
  | smiData.RevoluteJoint(30).Rz.Pos = -179.19615492437035;  % deg
  | smiData.RevoluteJoint(30).ID = '[Leg_Assembly_Y-P-6:Leg_part_05-1:-:Leg_Assembly_Y-P-6:Leg_part_04-1]';
undefined symbols (not defined in the file): density_ABS, mass_xm430, smiData, X, Y, Z
libraries: sm_lib x278, nesl_utility x39, Contact_Forces_Lib x12
(part 1 of 7)
settings Model: Creator=Kevin_Home  LastModifiedBy=kggim2

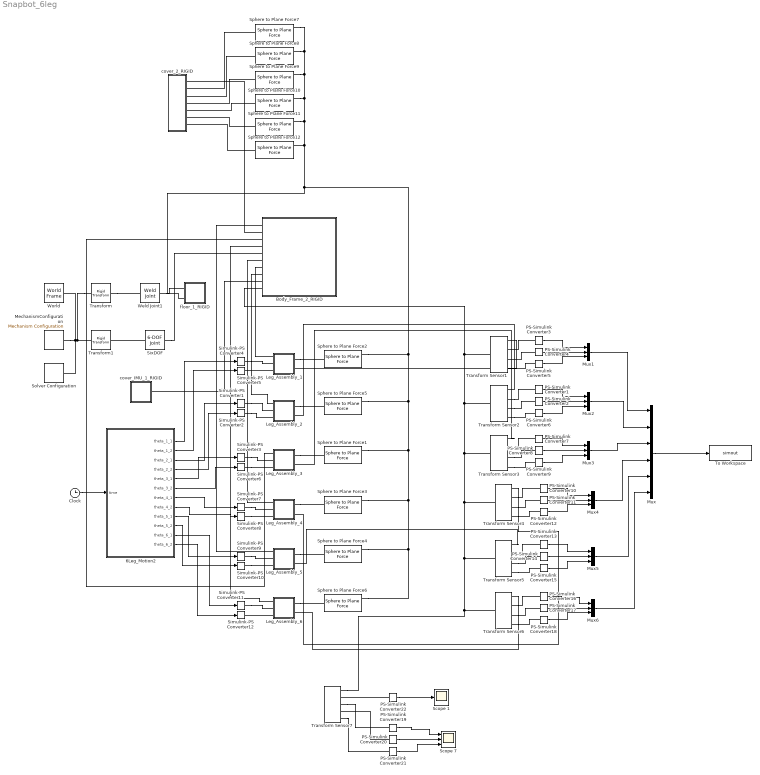
== system Snapbot_6leg ==
  6Leg_Motion2 : MATLAB Function  TreatAsAtomicUnit=on
  Body_Frame_2_RIGID : Subsystem
  Clock : Clock
  "Leg_Assembly_1 " : Subsystem
  Leg_Assembly_2 : Subsystem
  Leg_Assembly_3 : Subsystem
  Leg_Assembly_4 : Subsystem
  Leg_Assembly_5 : Subsystem
  Leg_Assembly_6 : Subsystem
  MechanismConfiguration : sm_lib/Utilities/Mechanism Configuration  UniformGravity=Constant  GravityVector="[0  0 -9.80665]"  GravityUnits=m/s^2  LinearizationDelta=0.001
  Mux : Mux  Inputs=6
  Mux{1..6} (6 alike) : Mux  Inputs=3
  PS-Simulink Converter{1..21} (21 alike) : nesl_utility/PS-Simulink Converter  PhysicalDomain=network_engine_domain  SubClassName=ps_output  LeftPortType=input  RightPortType=output  PseudoPeriodic=off  Frequencies=[]  Unit=mm  AffineConversion=off
  PS-Simulink Converter22 : nesl_utility/PS-Simulink Converter  PhysicalDomain=network_engine_domain  SubClassName=ps_output  LeftPortType=input  RightPortType=output  PseudoPeriodic=off  Frequencies=[]  Unit=rad  AffineConversion=off
  Scope 1 : Scope
  Scope 7 : Scope  NumInputPorts=3
  Simulink-PS Converter{1..12} (12 alike) : nesl_utility/Simulink-PS Converter  PhysicalDomain=network_engine_domain  SubClassName=ps_input  LeftPortType=input  RightPortType=output  PseudoPeriodic=off  Frequencies=[]  NoiseDistribution=none  NoiseParameters=[]  Unit=1  AffineConversion=off  FilteringAndDerivatives=filter  SimscapeFilterOrder=2  InputFilterTimeConstant=0.001  UdotUserProvided=0
  SixDOF : sm_lib/Joints/6-DOF Joint  JointMode=Normal  SenseConstraintForce=off  SenseConstraintForceX=off  SenseConstraintForceY=off  SenseConstraintForceZ=off  SenseConstraintTorque=off  SenseConstraintTorqueX=off  SenseConstraintTorqueY=off  SenseConstraintTorqueZ=off  SenseTotalForce=off  SenseTotalForceX=off  SenseTotalForceY=off  SenseTotalForceZ=off  SenseTotalTorque=off  SenseTotalTorqueX=off  SenseTotalTorqueY=off  SenseTotalTorqueZ=off  CompositeWrenchDir=FollowerOnBase  CompositeWrenchFrame=BaseFrame  PxEquilibriumPosition=0  PxEquilibriumPositionUnits=m  PxSpringStiffness=0  PxSpringStiffnessUnits=N/m  PxDampingCoefficient=0  PxDampingCoefficientUnits=N/(m/s)  PxTorqueActuationMode=NoTorque  PxMotionActuationMode=ComputedMotion  PxSensePosition=off  PxSenseVelocity=off  PxSenseAcceleration=off  PxSenseTorqueForce=off  PxSenseLowerLimitTorqueForce=off  PxSenseUpperLimitTorqueForce=off  PxLowerLimitSpecify=off  PxLowerLimitBound=-1  PxLowerLimitBoundUnits=m  PxLowerLimitStiffness=1e6  PxLowerLimitStiffnessUnits=N/m  PxLowerLimitDamping=1e3  PxLowerLimitDampingUnits=N/(m/s)  PxLowerLimitTransitionRegionWidth=1e-4  PxLowerLimitTransitionRegionWidthUnits=m  PxUpperLimitSpecify=off  PxUpperLimitBound=1  PxUpperLimitBoundUnits=m  PxUpperLimitStiffness=1e6  PxUpperLimitStiffnessUnits=N/m  PxUpperLimitDamping=1e3  PxUpperLimitDampingUnits=N/(m/s)  PxUpperLimitTransitionRegionWidth=1e-4  PxUpperLimitTransitionRegionWidthUnits=m  PxPositionTargetSpecify=off  PxPositionTargetPriority=High  PxPositionTargetValue=0  PxPositionTargetValueUnits=m  PxVelocityTargetSpecify=off  PxVelocityTargetPriority=High  PxVelocityTargetValue=0  PxVelocityTargetValueUnits=m/s  PyEquilibriumPosition=0  PyEquilibriumPositionUnits=m  PySpringStiffness=0  PySpringStiffnessUnits=N/m  PyDampingCoefficient=0  PyDampingCoefficientUnits=N/(m/s)  PyTorqueActuationMode=NoTorque  PyMotionActuationMode=ComputedMotion  PySensePosition=off  PySenseVelocity=off  PySenseAcceleration=off  PySenseTorqueForce=off  PySenseLowerLimitTorqueForce=off  PySenseUpperLimitTorqueForce=off  PyLowerLimitSpecify=off  PyLowerLimitBound=-1  PyLowerLimitBoundUnits=m  PyLowerLimitStiffness=1e6  PyLowerLimitStiffnessUnits=N/m  PyLowerLimitDamping=1e3  PyLowerLimitDampingUnits=N/(m/s)  PyLowerLimitTransitionRegionWidth=1e-4  PyLowerLimitTransitionRegionWidthUnits=m  PyUpperLimitSpecify=off  PyUpperLimitBound=1  PyUpperLimitBoundUnits=m  PyUpperLimitStiffness=1e6  PyUpperLimitStiffnessUnits=N/m  PyUpperLimitDamping=1e3  PyUpperLimitDampingUnits=N/(m/s)  PyUpperLimitTransitionRegionWidth=1e-4  PyUpperLimitTransitionRegionWidthUnits=m  PyPositionTargetSpecify=off  PyPositionTargetPriority=High  PyPositionTargetValue=0  PyPositionTargetValueUnits=m  PyVelocityTargetSpecify=off  PyVelocityTargetPriority=High  PyVelocityTargetValue=0  PyVelocityTargetValueUnits=m/s  PzEquilibriumPosition=0  PzEquilibriumPositionUnits=m  PzSpringStiffness=0  PzSpringStiffnessUnits=N/m  PzDampingCoefficient=0  PzDampingCoefficientUnits=N/(m/s)  PzTorqueActuationMode=NoTorque  PzMotionActuationMode=ComputedMotion  PzSensePosition=off  PzSenseVelocity=off  PzSenseAcceleration=off  PzSenseTorqueForce=off  PzSenseLowerLimitTorqueForce=off  PzSenseUpperLimitTorqueForce=off  PzLowerLimitSpecify=off  PzLowerLimitBound=-1  PzLowerLimitBoundUnits=m  PzLowerLimitStiffness=1e6  PzLowerLimitStiffnessUnits=N/m  PzLowerLimitDamping=1e3  PzLowerLimitDampingUnits=N/(m/s)  PzLowerLimitTransitionRegionWidth=1e-4  PzLowerLimitTransitionRegionWidthUnits=m  PzUpperLimitSpecify=off  PzUpperLimitBound=1  PzUpperLimitBoundUnits=m  PzUpperLimitStiffness=1e6  PzUpperLimitStiffnessUnits=N/m  PzUpperLimitDamping=1e3  PzUpperLimitDampingUnits=N/(m/s)  PzUpperLimitTransitionRegionWidth=1e-4  PzUpperLimitTransitionRegionWidthUnits=m  PzPositionTargetSpecify=off  PzPositionTargetPriority=High  PzPositionTargetValue=0  PzPositionTargetValueUnits=m  PzVelocityTargetSpecify=off  PzVelocityTargetPriority=High  PzVelocityTargetValue=0  PzVelocityTargetValueUnits=m/s  SphDefPosRotationMethod=None  SphDefPosRotationAngleUnits=deg  SphDefPosRotationStandardAxis=+Z  SphDefPosRotationAngle=0.0  SphDefPosRotationArbitraryAxis=[0 0 1]  SphDefPosFollAlignAxisA=+X  SphDefPosBaseAlignAxisA=+Y  SphDefPosFollAlignAxisB=+Y  SphDefPosBaseAlignAxisB=+Z  SphDefPosRotationSequenceAxes=FollowerAxes  SphDefPosRotationSequence=XYX  SphDefPosRotationSequenceAngles=[0 0 0]  SphDefPosRotationSequenceAnglesUnits=deg  SphDefPosRotationMatrix=[1 0 0; 0 1 0; 0 0 1]  SphEqPosRotationMethod=None  SphEqPosRotationAngleUnits=deg  SphEqPosRotationStandardAxis=+Z  SphEqPosRotationAngle=0.0  SphEqPosRotationArbitraryAxis=[0 0 1]  SphEqPosFollAlignAxisA=+X  SphEqPosBaseAlignAxisA=+Y  SphEqPosFollAlignAxisB=+Y  SphEqPosBaseAlignAxisB=+Z  SphEqPosRotationSequenceAxes=FollowerAxes  SphEqPosRotationSequence=XYX  SphEqPosRotationSequenceAngles=[0 0 0]  SphEqPosRotationSequenceAnglesUnits=deg  SphEqPosRotationMatrix=[1 0 0; 0 1 0; 0 0 1]  SphSpringStiffness=0  SphSpringStiffnessUnits=N*m/rad  SphDampingCoefficient=0  SphDampingCoefficientUnits=N*m/(rad/s)  SphActuateTorqueX=off  SphActuateTorqueY=off  SphActuateTorqueZ=off  SphActuateTorque=off  SphTorqueActuationMode=NoTorque  SphMotionActuationMode=ComputedMotion  SphActuationFrame=BaseFrame  SphSensePosition=off  SphSenseVelocityX=off  SphSenseVelocityY=off  SphSenseVelocityZ=off  SphSenseVelocity=off  SphSenseAccelerationX=off  SphSenseAccelerationY=off  SphSenseAccelerationZ=off  SphSenseAcceleration=off  SphSenseTorqueX=off  SphSenseTorqueY=off  SphSenseTorqueZ=off  SphSenseTorqueForce=off  SphSenseLowerLimitTorqueMag=off  SphSenseUpperLimitTorqueMag=off  SphSensingFrame=FollowerFrame  SphLowerLimitSpecify=off  SphLowerLimitBound=15  SphLowerLimitBoundUnits=deg  SphLowerLimitStiffness=1e4  SphLowerLimitStiffnessUnits=N*m/deg  SphLowerLimitDamping=10  SphLowerLimitDampingUnits=N*m/(deg/s)  SphLowerLimitTransitionRegionWidth=0.1  SphLowerLimitTransitionRegionWidthUnits=deg  SphUpperLimitSpecify=off  SphUpperLimitBound=45  SphUpperLimitBoundUnits=deg  SphUpperLimitStiffness=1e4  SphUpperLimitStiffnessUnits=N*m/deg  SphUpperLimitDamping=10  SphUpperLimitDampingUnits=N*m/(deg/s)  SphUpperLimitTransitionRegionWidth=0.1  SphUpperLimitTransitionRegionWidthUnits=deg  SphPositionTargetRotationMethod=None  SphPositionTargetRotationAngleUnits=deg  SphPositionTargetRotationStandardAxis=+Z  SphPositionTargetRotationAngle=0.0  SphPositionTargetRotationArbitraryAxis=[0 0 1]  SphPositionTargetFollAlignAxisA=+X  SphPositionTargetBaseAlignAxisA=+Y  SphPositionTargetFollAlignAxisB=+Y  SphPositionTargetBaseAlignAxisB=+Z  SphPositionTargetRotationSequenceAxes=FollowerAxes  SphPositionTargetRotationSequence=XYX  SphPositionTargetRotationSequenceAngles=[0 0 0]  SphPositionTargetRotationSequenceAnglesUnits=deg  SphPositionTargetRotationMatrix=[1 0 0; 0 1 0; 0 0 1]  SphPositionTargetSpecify=off  SphPositionTargetPriority=High  SphVelocityTargetValue=[0 0 0]  SphVelocityTargetValueUnits=deg/s  SphVelocityTargetSpecify=off  SphVelocityTargetPriority=High  SphVelocityTargetInFollowerFrame=on
  Solver Configuration : nesl_utility/Solver Configuration  PhysicalDomain=network_engine_domain  SubClassName=solver  LeftPortType=input  RightPortType=generic  Tones=[]  Harmonics=[]  SimulateNoise=off  Profile=off  UseLocalSampling=off  EnableSwitchedLinearOptims=on  FrequencyDomain=off  UseCCode=off  RelTol=0.001  AbsTol=1e-06  MinStep=1e-09  ToWorkspace=off  RevertToSquareIcSolve=off  NumHomotopyIterations=100  PhasorMode=off  PhasorModeNumHarmonics=1  DoDC=off  ResidualTolerance=1e-09  UseLocalSolver=off  LocalSolverChoice=NE_BACKWARD_EULER_ADVANCER  LocalSolverSampleTime=0.001  DoFixedCost=off  MaxNonlinIter=3  MaxModeIter=2  LinearAlgebra=auto  EquationFormulation=NE_TIME_EF  DelaysMemoryBudget=1024  AutomaticFiltering=on  FilteringTimeConstant=0.001  PartitionStorageMethod=AS_NEEDED  PartitionMemoryBudget=1024  PartitionMethod=ROBUST
  Sphere to Plane Force{1..5} (5 alike) : Contact_Forces_Lib/3D/Sphere to Plane Force  sphere_rad=Sphere_R_1  plane_lenx=Plane_x  plane_leny=Plane_y  plane_depth=Plane_d  force_law=Linear  k_contact=Contact_Stiff_1  b_contact=Contact_Damp_1  pen_full_damp_F=1e-4  pen_exponent=1  custom_param_1=1  custom_param_2=1  friction_law=Stick-Slip Continuous  mu_kinetic=Coff_KF_1  mu_static=Coff_SF_1  v_thr=Thres_Vel_1  vis_on=off  vis_opc_en=0  vis_len_plaBz=0.001  vis_clr=[0.9 0.2 0.2]  vis_opc=0.7
  Sphere to Plane Force{8..12} (5 alike) : Contact_Forces_Lib/3D/Sphere to Plane Force  sphere_rad=Sphere_R_2  plane_lenx=Plane_x  plane_leny=Plane_y  plane_depth=Plane_d  force_law=Linear  k_contact=Contact_Stiff_2  b_contact=Contact_Damp_2  pen_full_damp_F=1e-4  pen_exponent=1  custom_param_1=1  custom_param_2=1  friction_law=Stick-Slip Continuous  mu_kinetic=Coff_KF_2  mu_static=Coff_SF_2  v_thr=Thres_Vel_2  vis_on=off  vis_opc_en=0  vis_len_plaBz=0.005  vis_clr=[0.9 0.2 0.2]  vis_opc=0.7
  Sphere to Plane Force6 : Contact_Forces_Lib/3D/Sphere to Plane Force  sphere_rad=Sphere_R_1  plane_lenx=Plane_x  plane_leny=Plane_y  plane_depth=Plane_d  force_law=Linear  k_contact=Contact_Stiff_1  b_contact=Contact_Damp_1  pen_full_damp_F=1e-4  pen_exponent=1  custom_param_1=1  custom_param_2=1  friction_law=Stick-Slip Continuous  mu_kinetic=Coff_KF_1  mu_static=Coff_SF_1  v_thr=Thres_Vel_1  vis_on=on  vis_opc_en=0  vis_len_plaBz=0.005  vis_clr=[0.9 0.9 0.9]  vis_opc=0.7
  Sphere to Plane Force7 : Contact_Forces_Lib/3D/Sphere to Plane Force  sphere_rad=Sphere_R_2  plane_lenx=Plane_x  plane_leny=Plane_y  plane_depth=Plane_d  force_law=Linear  k_contact=Contact_Stiff_2  b_contact=Contact_Damp_2  pen_full_damp_F=1e-4  pen_exponent=1  custom_param_1=1  custom_param_2=1  friction_law=Stick-Slip Continuous  mu_kinetic=Coff_KF_2  mu_static=Coff_SF_2  v_thr=Thres_Vel_2  vis_on=off  vis_opc_en=0  vis_len_plaBz=0.0001  vis_clr=[0.9 0.2 0.2]  vis_opc=0.7
  To Workspace : ToWorkspace  VariableName=simout  SaveFormat=Timeseries  SampleTime=-1
  Transform : sm_lib/Frames and Transforms/Rigid Transform  TranslationMethod=Cartesian  TranslationStandardOffset=0  TranslationLengthUnit=mm  TranslationStandardAxis=+Z  TranslationCartesianOffset=smiData.RigidTransform(24).translation-[0 0 1.5]  TranslationROffset=0  TranslationROffsetUnits=m  TranslationZOffset=0  TranslationZOffsetUnits=m  TranslationThetaOffset=0  TranslationThetaOffsetUnits=deg  RotationMethod=ArbitraryAxis  RotationAngleUnits=rad  RotationStandardAxis=+Z  RotationAngle=smiData.RigidTransform(24).angle  RotationArbitraryAxis=smiData.RigidTransform(24).axis  FollAlignAxisA=+X  BaseAlignAxisA=+Y  FollAlignAxisB=+Y  BaseAlignAxisB=+Z  RotationSequenceAxes=FollowerAxes  RotationSequence=XYX  RotationSequenceAngles=[0 0 0]  RotationSequenceAnglesUnits=deg  RotationMatrix=[1 0 0; 0 1 0; 0 0 1]
  Transform Sensor{1..6} (6 alike) : sm_lib/Frames and Transforms/Transform Sensor  MeasurementFrame=Base  SenseAngle=off  SenseAxis=off  SenseAngle1=off  SenseAngle2=off  SenseAngle3=off  SenseQ=off  SenseR=off  SenseOmegaX=off  SenseOmegaY=off  SenseOmegaZ=off  SenseOmega1=off  SenseOmega2=off  SenseOmega3=off  SenseQDot=off  SenseRDot=off  SenseAlphaX=off  SenseAlphaY=off  SenseAlphaZ=off  SenseAlpha1=off  SenseAlpha2=off  SenseAlpha3=off  SenseQDDot=off  SenseRDDot=off  SenseX=on  SenseY=on  SenseZ=on  SenseRad=off  SenseAzim=off  SenseDist=off  SenseInc=off  SenseXDot=off  SenseYDot=off  SenseZDot=off  SenseRadDot=off  SenseAzimDot=off  SenseDistDot=off  SenseIncDot=off  SenseXDDot=off  SenseYDDot=off  SenseZDDot=off  SenseRadDDot=off  SenseAzimDDot=off  SenseDistDDot=off  SenseIncDDot=off
  Transform Sensor7 : sm_lib/Frames and Transforms/Transform Sensor  MeasurementFrame=World  SenseAngle=on  SenseAxis=off  SenseAngle1=off  SenseAngle2=off  SenseAngle3=off  SenseQ=off  SenseR=off  SenseOmegaX=off  SenseOmegaY=off  SenseOmegaZ=off  SenseOmega1=off  SenseOmega2=off  SenseOmega3=off  SenseQDot=off  SenseRDot=off  SenseAlphaX=off  SenseAlphaY=off  SenseAlphaZ=off  SenseAlpha1=off  SenseAlpha2=off  SenseAlpha3=off  SenseQDDot=off  SenseRDDot=off  SenseX=on  SenseY=on  SenseZ=on  SenseRad=off  SenseAzim=off  SenseDist=off  SenseInc=off  SenseXDot=off  SenseYDot=off  SenseZDot=off  SenseRadDot=off  SenseAzimDot=off  SenseDistDot=off  SenseIncDot=off  SenseXDDot=off  SenseYDDot=off  SenseZDDot=off  SenseRadDDot=off  SenseAzimDDot=off  SenseDistDDot=off  SenseIncDDot=off
  Transform1 : sm_lib/Frames and Transforms/Rigid Transform  TranslationMethod=Cartesian  TranslationStandardOffset=0  TranslationLengthUnit=mm  TranslationStandardAxis=+Z  TranslationCartesianOffset=smiData.RigidTransform(41).translation  TranslationROffset=0  TranslationROffsetUnits=m  TranslationZOffset=0  TranslationZOffsetUnits=m  TranslationThetaOffset=0  TranslationThetaOffsetUnits=deg  RotationMethod=ArbitraryAxis  RotationAngleUnits=rad  RotationStandardAxis=+Z  RotationAngle=smiData.RigidTransform(41).angle  RotationArbitraryAxis=smiData.RigidTransform(41).axis  FollAlignAxisA=+X  BaseAlignAxisA=+Y  FollAlignAxisB=+Y  BaseAlignAxisB=+Z  RotationSequenceAxes=FollowerAxes  RotationSequence=XYX  RotationSequenceAngles=[0 0 0]  RotationSequenceAnglesUnits=deg  RotationMatrix=[1 0 0; 0 1 0; 0 0 1]
  Weld Joint1 : sm_lib/Joints/Weld Joint  JointMode=Normal  SenseConstraintForce=off  SenseConstraintForceX=off  SenseConstraintForceY=off  SenseConstraintForceZ=off  SenseConstraintTorque=off  SenseConstraintTorqueX=off  SenseConstraintTorqueY=off  SenseConstraintTorqueZ=off  SenseTotalForce=off  SenseTotalForceX=off  SenseTotalForceY=off  SenseTotalForceZ=off  SenseTotalTorque=off  SenseTotalTorqueX=off  SenseTotalTorqueY=off  SenseTotalTorqueZ=off  CompositeWrenchDir=FollowerOnBase  CompositeWrenchFrame=BaseFrame
  World : sm_lib/Frames and Transforms/World Frame
  cover_2_RIGID : Subsystem
  cover_IMU_1_RIGID : Subsystem
  floor_1_RIGID : Subsystem
  wires:
  Clock/1 -> 6Leg_Motion2/1(time)
  6Leg_Motion2/1(theta_1_1) -> Simulink-PS Converter4/1
  6Leg_Motion2/2(theta_1_2) -> Simulink-PS Converter5/1
  6Leg_Motion2/3(theta_2_1) -> Simulink-PS Converter1/1
  6Leg_Motion2/4(theta_2_2) -> Simulink-PS Converter2/1
  6Leg_Motion2/5(theta_3_1) -> Simulink-PS Converter3/1
  6Leg_Motion2/6(theta_3_2) -> Simulink-PS Converter6/1
  6Leg_Motion2/7(theta_4_1) -> Simulink-PS Converter7/1
  6Leg_Motion2/8(theta_4_2) -> Simulink-PS Converter8/1
  6Leg_Motion2/9(theta_5_1) -> Simulink-PS Converter9/1
  6Leg_Motion2/10(theta_5_2) -> Simulink-PS Converter10/1
  6Leg_Motion2/11(theta_6_1) -> Simulink-PS Converter11/1
  6Leg_Motion2/12(theta_6_2) -> Simulink-PS Converter12/1
  PS-Simulink Converter4/1 -> Mux1/2
  PS-Simulink Converter3/1 -> Mux1/1
  PS-Simulink Converter5/1 -> Mux1/3
  PS-Simulink Converter1/1 -> Mux2/1
  PS-Simulink Converter2/1 -> Mux2/2
  PS-Simulink Converter6/1 -> Mux2/3
  PS-Simulink Converter8/1 -> Mux3/2
  PS-Simulink Converter7/1 -> Mux3/1
  PS-Simulink Converter9/1 -> Mux3/3
  PS-Simulink Converter11/1 -> Mux4/2
  PS-Simulink Converter10/1 -> Mux4/1
  PS-Simulink Converter12/1 -> Mux4/3
  PS-Simulink Converter14/1 -> Mux5/2
  PS-Simulink Converter13/1 -> Mux5/1
  PS-Simulink Converter15/1 -> Mux5/3
  PS-Simulink Converter17/1 -> Mux6/2
  PS-Simulink Converter16/1 -> Mux6/1
  PS-Simulink Converter18/1 -> Mux6/3
  Mux/1 -> To Workspace/1
  PS-Simulink Converter19/1 -> Scope 7/1
  PS-Simulink Converter20/1 -> Scope 7/2
  PS-Simulink Converter21/1 -> Scope 7/3
  Mux6/1 -> Mux/6
  Mux5/1 -> Mux/5
  Mux4/1 -> Mux/4
  Mux3/1 -> Mux/3
  Mux2/1 -> Mux/2
  Mux1/1 -> Mux/1
  PS-Simulink Converter22/1 -> Scope 1/1
  connections:
  Transform/LConn1 -- MechanismConfiguration/RConn1 -- Solver Configuration/RConn1 -- World/RConn1 -- Transform1/LConn1
  Body_Frame_2_RIGID/LConn9 -- cover_IMU_1_RIGID/LConn1
  SixDOF/RConn1 -- Body_Frame_2_RIGID/LConn5
  SixDOF/LConn1 -- Transform1/RConn1
  Body_Frame_2_RIGID/LConn8 -- Leg_Assembly_2/LConn1
  Body_Frame_2_RIGID/LConn7 -- "Leg_Assembly_1 "/LConn1
  Weld Joint1/RConn1 -- floor_1_RIGID/LConn1
  Body_Frame_2_RIGID/LConn6 -- Leg_Assembly_4/LConn1
  Body_Frame_2_RIGID/LConn4 -- Leg_Assembly_6/LConn1
  Body_Frame_2_RIGID/LConn3 -- Leg_Assembly_3/LConn1
  Body_Frame_2_RIGID/LConn2 -- cover_2_RIGID/LConn1
  Body_Frame_2_RIGID/LConn1 -- Leg_Assembly_5/LConn1
  Sphere to Plane Force7/LConn1 -- cover_2_RIGID/LConn2
  Sphere to Plane Force8/LConn1 -- cover_2_RIGID/LConn3
  Sphere to Plane Force11/LConn1 -- cover_2_RIGID/LConn6
  Sphere to Plane Force10/LConn1 -- cover_2_RIGID/LConn5
  Sphere to Plane Force9/LConn1 -- cover_2_RIGID/LConn4
  Sphere to Plane Force12/LConn1 -- cover_2_RIGID/LConn7
  floor_1_RIGID/LConn2 -- Sphere to Plane Force5/RConn1 -- Sphere to Plane Force1/RConn1 -- Sphere to Plane Force6/RConn1 -- Sphere to Plane Force4/RConn1 -- Sphere to Plane Force3/RConn1 -- Sphere to Plane Force2/RConn1 -- Sphere to Plane Force7/RConn1 -- Sphere to Plane Force8/RConn1 -- Sphere to Plane Force9/RConn1 -- Sphere to Plane Force10/RConn1 -- Sphere to Plane Force11/RConn1 -- Sphere to Plane Force12/RConn1
  Transform/RConn1 -- Weld Joint1/LConn1
  "Leg_Assembly_1 "/RConn1 -- Sphere to Plane Force2/LConn1
  Leg_Assembly_4/RConn1 -- Sphere to Plane Force3/LConn1
  Leg_Assembly_3/RConn1 -- Sphere to Plane Force1/LConn1
  Leg_Assembly_6/RConn1 -- Sphere to Plane Force6/LConn1
  Leg_Assembly_5/RConn1 -- Sphere to Plane Force4/LConn1
  Leg_Assembly_2/RConn1 -- Sphere to Plane Force5/LConn1
  Simulink-PS Converter4/RConn1 -- "Leg_Assembly_1 "/LConn2
  "Leg_Assembly_1 "/LConn3 -- Simulink-PS Converter5/RConn1
  Simulink-PS Converter1/RConn1 -- Leg_Assembly_2/LConn2
  Simulink-PS Converter2/RConn1 -- Leg_Assembly_2/LConn3
  Simulink-PS Converter3/RConn1 -- Leg_Assembly_3/LConn2
  Simulink-PS Converter6/RConn1 -- Leg_Assembly_3/LConn3
  Simulink-PS Converter7/RConn1 -- Leg_Assembly_4/LConn2
  Simulink-PS Converter8/RConn1 -- Leg_Assembly_4/LConn3
  Simulink-PS Converter9/RConn1 -- Leg_Assembly_5/LConn2
  Simulink-PS Converter10/RConn1 -- Leg_Assembly_5/LConn3
  Simulink-PS Converter11/RConn1 -- Leg_Assembly_6/LConn2
  Leg_Assembly_6/LConn3 -- Simulink-PS Converter12/RConn1
  Transform Sensor1/RConn4 -- PS-Simulink Converter5/LConn1
  Transform Sensor1/RConn2 -- PS-Simulink Converter3/LConn1
  Transform Sensor1/RConn1 -- "Leg_Assembly_1 "/RConn2
  Transform Sensor1/RConn3 -- PS-Simulink Converter4/LConn1
  Body_Frame_2_RIGID/LConn10 -- Transform Sensor6/LConn1 -- Transform Sensor7/RConn1 -- Transform Sensor5/LConn1 -- Transform Sensor4/LConn1 -- Transform Sensor3/LConn1 -- Transform Sensor2/LConn1 -- Transform Sensor1/LConn1
  Transform Sensor2/RConn2 -- PS-Simulink Converter1/LConn1
  Transform Sensor2/RConn1 -- Leg_Assembly_2/RConn2
  Transform Sensor2/RConn3 -- PS-Simulink Converter2/LConn1
  Transform Sensor2/RConn4 -- PS-Simulink Converter6/LConn1
  Transform Sensor3/RConn4 -- PS-Simulink Converter9/LConn1
  Transform Sensor3/RConn2 -- PS-Simulink Converter7/LConn1
  Transform Sensor3/RConn1 -- Leg_Assembly_3/RConn2
  Transform Sensor3/RConn3 -- PS-Simulink Converter8/LConn1
  Transform Sensor4/RConn4 -- PS-Simulink Converter12/LConn1
  Transform Sensor4/RConn2 -- PS-Simulink Converter10/LConn1
  Transform Sensor4/RConn1 -- Leg_Assembly_4/RConn2
  Transform Sensor4/RConn3 -- PS-Simulink Converter11/LConn1
  Transform Sensor5/RConn4 -- PS-Simulink Converter15/LConn1
  Transform Sensor5/RConn2 -- PS-Simulink Converter13/LConn1
  Transform Sensor5/RConn1 -- Leg_Assembly_5/RConn2
  Transform Sensor5/RConn3 -- PS-Simulink Converter14/LConn1
  Transform Sensor6/RConn4 -- PS-Simulink Converter18/LConn1
  Transform Sensor6/RConn2 -- PS-Simulink Converter16/LConn1
  Transform Sensor6/RConn1 -- Leg_Assembly_6/RConn2
  Transform Sensor6/RConn3 -- PS-Simulink Converter17/LConn1
  Transform Sensor7/RConn3 -- PS-Simulink Converter19/LConn1
  PS-Simulink Converter20/LConn1 -- Transform Sensor7/RConn4
  Transform Sensor7/RConn5 -- PS-Simulink Converter21/LConn1
  PS-Simulink Converter22/LConn1 -- Transform Sensor7/RConn2
